simulink model "model2"  (R2015a)
settings: Solver=ode4  StartTime=0.0  StopTime=20.0  FixedStep=0.01  RelTol=1e-3
settings Model: Creator=jleny  LastModifiedBy=jleny

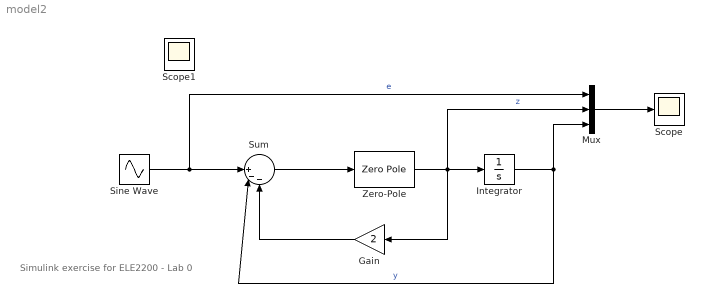
== system model2 ==
  note: Simulink exercise for ELE2200 - Lab 0
  Gain : Gain  Gain=2
  Integrator : Integrator
  Mux : Mux  Inputs=3
  Scope : Scope
  Sine Wave : Sin  Amplitude=0.1  Bias=1  Frequency=5  SampleTime=0
  Sum : Sum  Inputs=||+--
  Zero-Pole : ZeroPole  Zeros=[-5]  Poles=[0 -10]  Gain=[2]
  Scope1 : Scope
  wires:
  Sine Wave/1 -> Mux/1, Sum/1  "e"
  Zero-Pole/1 -> Mux/2, Gain/1, Integrator/1  "z"
  Gain/1 -> Sum/3
  Sum/1 -> Zero-Pole/1
  Integrator/1 -> Sum/2, Mux/3  "y"
  Mux/1 -> Scope/1
